simulink model "simu"  (R2022b)
settings: Solver=FixedStepAuto  StartTime=0.0  StopTime=t_max  FixedStep=timestep  RelTol=1e-3
values from neighbouring files (symbols this model uses):
  Kae = 1    [script.m]
  Kdg = 1    [script.m]
  Kf = 1    [script.m]
  Kp = 2    [script.m]
  Ku = 0.4    [script.m]
  Kwt = 1    [script.m]
  step_v = 100    [script.m]
  Tae = 0.2    [script.m]
  Td = 0.024    [script.m]
  Tdg = 2    [script.m]
  Tf = 4    [script.m]
  timestep = t_max/1e6    (= 1e-06)    [script.m]
  Tp = 20    [script.m]
  Twt = 1.5    [script.m]
libraries: simulink x1
settings Model: Creator=mluser  LastModifiedBy=mluser

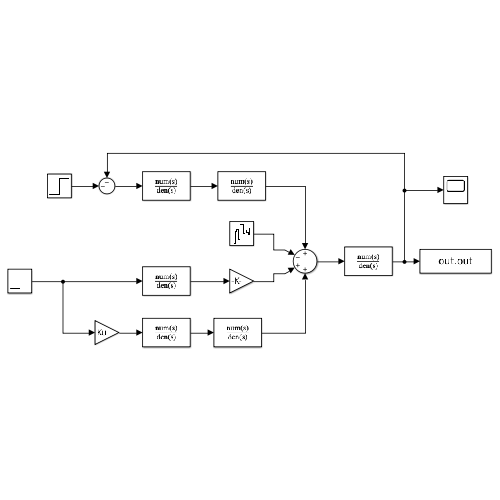
[thumbnail: Simulink's stored preview of the top-level diagram]
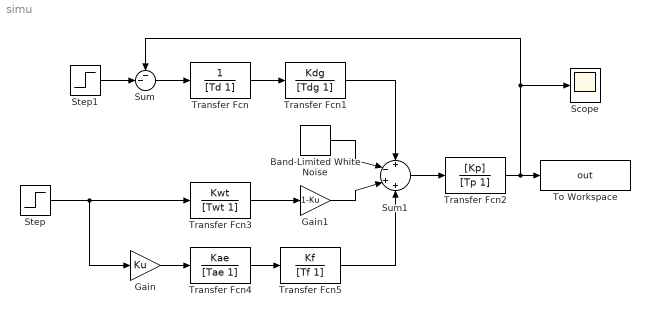
== system simu ==
  Band-Limited White Noise : simulink/Sources/Band-Limited White Noise  Cov=random_power  Ts=timestep  seed=[23341]
  Gain : Gain  Gain=Ku
  Gain1 : Gain  Gain=1-Ku
  Scope : Scope
  Step : Step  Time=step_v  SampleTime=0
  Step1 : Step  SampleTime=0
  Sum : Sum  Inputs=--|
  Sum1 : Sum  Inputs=+-++
  To Workspace : ToWorkspace  VariableName=out  SampleTime=-1
  Transfer Fcn : TransferFcn  Denominator=[Td 1]
  Transfer Fcn1 : TransferFcn  Numerator=Kdg  Denominator=[Tdg 1]
  Transfer Fcn2 : TransferFcn  Numerator=[Kp]  Denominator=[Tp 1]
  Transfer Fcn3 : TransferFcn  Numerator=Kwt  Denominator=[Twt 1]
  Transfer Fcn4 : TransferFcn  Numerator=Kae  Denominator=[Tae 1]
  Transfer Fcn5 : TransferFcn  Numerator=Kf  Denominator=[Tf 1]
  wires:
  Step1/1 -> Sum/2
  Transfer Fcn/1 -> Transfer Fcn1/1
  Sum/1 -> Transfer Fcn/1
  Transfer Fcn1/1 -> Sum1/1
  Band-Limited White Noise/1 -> Sum1/2
  Sum1/1 -> Transfer Fcn2/1
  Transfer Fcn2/1 -> To Workspace/1, Sum/1, Scope/1
  Step/1 -> Transfer Fcn3/1, Gain/1
  Gain1/1 -> Sum1/3
  Transfer Fcn3/1 -> Gain1/1
  Gain/1 -> Transfer Fcn4/1
  Transfer Fcn4/1 -> Transfer Fcn5/1
  Transfer Fcn5/1 -> Sum1/4
